simulink model "FIR_Filter0"  (R2020b)
settings: Solver=FixedStepAuto  StartTime=0.0  StopTime=10  FixedStep=0.2  RelTol=1e-3
settings Model: Creator=Manasi  LastModifiedBy=Manasi
settings DataIOCC: SaveOutput=off  SaveTime=off

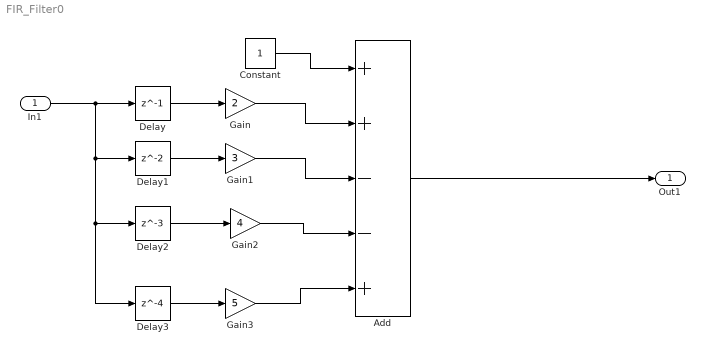
== system FIR_Filter0 ==
  In1 : Inport  OutDataTypeStr=double  PortDimensions=1  SampleTime=[0,1]
  Add : Sum  Inputs=++--+
  Constant : Constant
  Delay : Delay  DelayLength=1
  Delay1 : Delay
  Delay2 : Delay  DelayLength=3
  Delay3 : Delay  DelayLength=4
  Gain : Gain  Gain=2
  Gain1 : Gain  Gain=3
  Gain2 : Gain  Gain=4
  Gain3 : Gain  Gain=5
  Out1 : Outport  OutDataTypeStr=double  PortDimensions=1  SampleTime=[0.20000000000000001,0]
  wires:
  Gain3/1 -> Add/5
  In1/1 -> Delay/1, Delay1/1, Delay2/1, Delay3/1
  Delay2/1 -> Gain2/1
  Gain/1 -> Add/2
  Gain2/1 -> Add/4
  Delay/1 -> Gain/1
  Gain1/1 -> Add/3
  Constant/1 -> Add/1
  Delay1/1 -> Gain1/1
  Delay3/1 -> Gain3/1
  Add/1 -> Out1/1
